simulink model "termicos"  (Simulink 6.0)
settings: Solver=ode45  StartTime=0.0  StopTime=120  FixedStep=0.5  RelTol=1e-3
undefined symbols (not defined in the file or in its folder): a, b, c, d
settings Model: CovMetricSettings=we  CovNameIncrementing=on  CovHtmlReporting=off  covSaveCumulativeToWorkspaceVar=off  LastModifiedBy=Y  ExtModeTrigDuration=5000
settings DataIOCC: LimitDataPoints=off  MaxDataPoints=5000  SaveFormat=StructureWithTime  SignalLoggingName=sigsOut
settings OptimizationCC: BlockReduction=off  BooleanDataType=off  InlineInvariantSignals=off
settings DebuggingCC: SolverPrmCheckMsg=none
settings RTWCC: SystemTargetFile=rtwin.tlc  TemplateMakefile=rtwin.tmf  Description=Real-Time Windows Target  ProcessScript=rtwin_make_rtw_hook
settings RTWinTargetCC: TargetFcnLib=ansi_tfl_tmw.mat  GenFloatMathFcnCalls=ANSI_C  ModelReferenceCompliant=off  CCOptimize=on

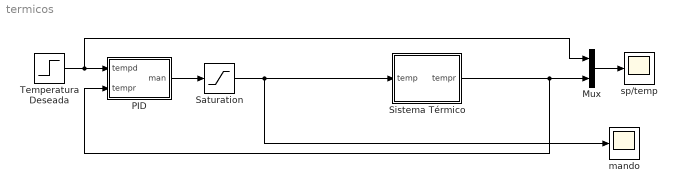
== system termicos ==
  Mux : Mux  Inputs=2
  PID : Subsystem  mask{kp=a, ki=b, kd=c}
  Saturation : Saturate  UpperLimit=10  LowerLimit=0
  Sistema Térmico : Subsystem
  Temperatura Deseada : Step  Time=0  After=d  SampleTime=0
  mando : Scope
      settings: TickLabels=on  YMin=4.75  YMax=8.75  SaveName=man  DataFormat=Array
  sp/temp : Scope
      settings: TickLabels=on  YMin=0  SaveName=temp  DataFormat=Array
  wires:
  Mux/1 -> sp/temp/1
  Temperatura Deseada/1 -> Mux/1, PID/1(tempd)
  PID/1(man) -> Saturation/1
  Saturation/1 -> mando/1, Sistema Térmico/1(temp)
  Sistema Térmico/1(tempr) -> Mux/2, PID/2(tempr)

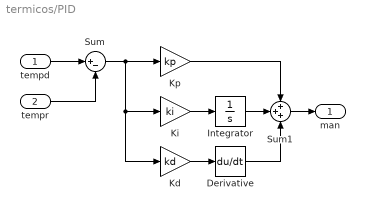
== system termicos/PID ==
  tempd : Inport  Port=1  LatchInput=off
  tempr : Inport  Port=2  LatchInput=off
  Derivative : Derivative
  Integrator : Integrator
  Kd : Gain  Gain=kd  SaturateOnIntegerOverflow=on
  Ki : Gain  Gain=ki  SaturateOnIntegerOverflow=on
  Kp : Gain  Gain=kp  SaturateOnIntegerOverflow=on
  Sum : Sum  Inputs=|+-  SaturateOnIntegerOverflow=on  InputSameDT=on
  Sum1 : Sum  Inputs=+++  SaturateOnIntegerOverflow=on  InputSameDT=on
  man : Outport
  wires:
  tempd/1 -> Sum/1
  tempr/1 -> Sum/2
  Sum/1 -> Kp/1, Ki/1, Kd/1
  Ki/1 -> Integrator/1
  Kd/1 -> Derivative/1
  Integrator/1 -> Sum1/2
  Derivative/1 -> Sum1/3
  Kp/1 -> Sum1/1
  Sum1/1 -> man/1

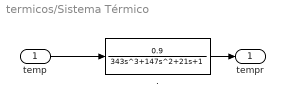
== system termicos/Sistema Térmico ==
  temp : Inport  Port=1  LatchInput=off
  . : TransferFcn  Numerator=0.9  Denominator="[343   147    21     1]"
  tempr : Outport
  wires:
  ./1 -> tempr/1
  temp/1 -> ./1
